simulink model "Model3Dpyhton"  (R2020a)
settings: Solver=VariableStepAuto  StartTime=0.0  StopTime=inf  FixedStep=0.2  RelTol=1e-3
model workspace (MAT data in the model file):
  VEH.Mass = 1181
  VEH.StaticNormalFrontLoad.FR = 264.666666667
  VEH.StaticNormalFrontLoad.FL = 264.666666667
  VEH.StaticNormalRearLoad.RR = 322
  VEH.StaticNormalRearLoad.RL = 322
  VEH.WheelBase = 3.075
  VEH.FrontAxlePositionfromCG = 1.515
  VEH.RearAxlePositionfromCG = 1.504
  VEH.HeightCG = 0.134
  VEH.FrontalArea = 2.11
  VEH.DragCoefficient = 0.33
  VEH.NumberOfWheelsPerAxle = 2
  VEH.Thread.FR = 1.705
  VEH.Thread.RR = 1.705
  VEH.PitchMomentInertia = 1922.66666667
  VEH.RollMomentInertia = 432.333333333
  VEH.YawMomentInertia = 2066
  VEH.SteeringRatio = 18
  VEH.TrackWidth = 1.922
  VEH.SprungMass = 1096.72266667
  VEH.InitialLongPosition = 0
  VEH.InitialLatPosition = 3.125
  VEH.InitialVertPosition = 0.0111
  VEH.InitialRollAngle = 0
  VEH.InitialPitchAngle = -0.000732
  VEH.InitialYawAngle = 0
  VEH.InitialLongVel = 0
  VEH.InitialLatVel = 0
  VEH.InitialVertVel = 0
  VEH.InitialRollRate = 0
  VEH.InitialPitchRate = 0
  VEH.InitialYawRate = 0
  color.orange = [1 0.6 0]
  color.red = [1 0.2 0]
  color.dgreen = [0 0.4 0]
  color.green = [0 0.6 0]
  color.lgreen = [0 0.8 0]
  color.dblue = [0 0.2 1]
  color.blue = [0.2 0.6 1]
  color.lblue = [0.4 0.8 1]
  color.brown = [0.4 0.2 0]
  color.lbrown = [0.8 0.4 0]
  color.yellow = [1 0.8 0]
  color.lyellow = [1 1 0]
  color.black = [0 0 0]
  color.white = [1 1 1]
  color.dgrey = [0.3 0.3 0.3]
  color.grey = [0.5 0.5 0.5]
  color.lgrey = [0.7 0.7 0.7]
  color.vlgrey = [0.9 0.9 0.9]
  cosAngle = 1
  density.wood = 650
  density.plastic = 920
  density.water = 1000
  density.aluminum = 2700
  density.steel = 7800
  density.titanium = 4500
  density.brass = 8600
  dwb.knuckle.height = 43
  dwb.knuckle.length = 8
  dwb.knuckle.thickness = 1
  dwb.knuckle.wheelattachprojwidth = 2.5
  dwb.knuckle.wheelattachprojheight = 8
  dwb.knuckle.wishboneconnectorwidth = 10
  dwb.knuckle.driveshaftradius = 2.5
  dwb.knuckle.driveshaftheight = 6
  dwb.knuckle.chamferradius = 0.25
  dwb.knuckle.transitionradius = 2
  dwb.knuckle.density = 2700
  dwb.knuckle.color = [0.3 0.3 0.3]
  dwb.knuckle.ball.radius = 1
  dwb.knuckle.pin.radius = 0.5
  dwb.knuckle.pin.height = 3
  dwb.knuckle.steerarm.length = 20
  dwb.knuckle.steerarm.width = 2
  dwb.knuckle.steerarm.thickness = 1
  dwb.knuckle.steerarm.forkheight = 13
  dwb.knuckle.steerarm.forklength = 4
  dwb.knuckle.steerarm.forkoffset = 3
  dwb.knuckle.pinradius = 0.25
  dwb.uwb.longlength = 25
  dwb.uwb.shortlength = 15
  dwb.uwb.wheellinklength = 5
  dwb.uwb.wheellinkwidth = 5
  dwb.uwb.width = 25
  dwb.uwb.thickness = 2
  dwb.uwb.baseradius = 8
  dwb.uwb.basearcoffset = 5
  dwb.uwb.density = 2700
  dwb.uwb.color = [0.3 0.2 0]
  dwb.uwb.bracket.length = 4
  dwb.uwb.bracket.radius = 0.75
  dwb.uwb.socket.radius = 2
  dwb.uwb.socket.height = 1.4
  dwb.uwb.socket.ballradius = 1
  dwb.uwb.socket.offset = 3
  dwb.lwb.longlength = 36
  dwb.lwb.shortlength = 25
  dwb.lwb.wheellinklength = 5
  dwb.lwb.wheellinkwidth = 5
  dwb.lwb.width = 14.75
  dwb.lwb.thickness = 2
  dwb.lwb.baseradius = 2.875
  dwb.lwb.basearcoffset = 15
  dwb.lwb.density = 2700
  dwb.lwb.color = [0.654901960784 0.423529411765 0.203921568627]
  dwb.lwb.bracket.length = 4
  dwb.lwb.bracket.radius = 0.75
  dwb.lwb.socket.radius = 2
  dwb.lwb.socket.height = 1.4
  dwb.lwb.socket.holeradius = 1
  dwb.lwb.socket.holeoffset = 3.0625
  dwb.lwb.damperbracket.offset = 10
  dwb.lwb.damperbracket.width = 4
  dwb.lwb.damperbracket.length = 4
  dwb.lwb.damperbracket.thickness = 1
  dwb.lwb.damperbracket.spacing = 1.5
  dwb.lwb.damperbracket.holeradius = 1
  dwb.springdamp.k = 100000
  dwb.springdamp.b = 11000
  dwb.springdamp.length0 = 18.5
  dwb.springdamp.density = 2700
  dwb.springdamp.cylinder.length = 22
  dwb.springdamp.cylinder.innerradius = 2
  dwb.springdamp.cylinder.outerradius = 3
  dwb.springdamp.cylinder.color = [0.9 0.7 0.2]
  dwb.springdamp.piston.length = 16
  dwb.springdamp.piston.color = [0.3 0.2 0]
  dwb.springdamp.chamferradius = 0.3
  dwb.springdamp.bracket.length = 6
  dwb.springdamp.bracket.width = 4
  dwb.springdamp.bracket.thickness = 1
  dwb.springdamp.bracket.holeradius = 0.75
  dwb.chassis.frame.longlength = 100
  dwb.chassis.frame.shortlength = 75
  dwb.chassis.frame.height = 40
  dwb.chassis.frame.cornerradius = 2
  dwb.chassis.frame.thickness = 2
  dwb.chassis.frame.barthickness = 5
  dwb.chassis.frame.density = 2700
  dwb.chassis.frame.color = [1 0.549019607843 0]
  dwb.chassis.upperlink.length = 30
  dwb.chassis.upperlink.outerradius = 1.5
  dwb.chassis.upperlink.innerradius = 0.75
  dwb.chassis.upperlink.wishboneslotlength = 5.5
  dwb.chassis.upperlink.springdamperslotlength = 3
  dwb.chassis.upperlink.wishboneseparation = 20.5
  dwb.chassis.upperlink.wishboneoffset = 0
  dwb.chassis.upperlink.chamferradius = 0.2
  dwb.chassis.upperlink.density = 2700
  dwb.chassis.upperlink.color = [1 0.549019607843 0]
  dwb.chassis.lowerlink.length = 30
  dwb.chassis.lowerlink.outerradius = 1.5
  dwb.chassis.lowerlink.innerradius = 0.75
  dwb.chassis.lowerlink.wishboneslotlength = 5.5
  dwb.chassis.lowerlink.wishboneseparation = 10.25
  dwb.chassis.lowerlink.wishboneoffset = 5.125
  dwb.chassis.lowerlink.chamferradius = 0.2
  dwb.chassis.lowerlink.density = 2700
  dwb.chassis.lowerlink.color = [1 0.549019607843 0]
  dwb.chassis.steering.bracket.length = 4
  dwb.chassis.steering.bracket.width = 4
  dwb.chassis.steering.bracket.thickness = 4
  dwb.chassis.steering.bracket.holelength = 2
  dwb.chassis.steering.bracket.holewidth = 2
  dwb.chassis.steering.bracket.chamferradius = 0.5
  dwb.chassis.steering.bracket.density = 2700
  dwb.chassis.steering.bracket.color = [1 0.549019607843 0]
  dwb.chassis.steering.tierod.rod.length = 16.5
  dwb.chassis.steering.tierod.rod.radius = 1.25
  dwb.chassis.steering.tierod.rod.chamferradius = 0.25
  dwb.chassis.steering.tierod.rod.color = [0.9 0.7 0.2]
  dwb.chassis.steering.tierod.bracket.length = 3
  dwb.chassis.steering.tierod.bracket.width = 2
  dwb.chassis.steering.tierod.bracket.thickness = 0.5
  dwb.chassis.steering.tierod.bracket.flangespacing = 0.75
  dwb.chassis.steering.tierod.bracket.socketradius = 0.75
  dwb.chassis.steering.tierod.bracket.ballradius = 0.5
  dwb.chassis.steering.tierod.bracket.holeradius = 0.3
  dwb.chassis.steering.tierod.density = 2700
  dwb.chassis.steering.tierod.ballcolor = [0.3 0.2 0]
  dwb.chassis.steering.rack.rod.length = 120
  dwb.chassis.steering.rack.rod.width = 2
  dwb.chassis.steering.rack.rod.height = 2
  dwb.chassis.steering.rack.rod.bracketdistance = 70
  dwb.chassis.steering.rack.rod.chamferradius = 0.5
  dwb.chassis.steering.rack.bracket.length = 4
  dwb.chassis.steering.rack.bracket.width = 2
  dwb.chassis.steering.rack.bracket.thickness = 0.5
  dwb.chassis.steering.rack.bracket.holeradius = 0.5
  dwb.chassis.steering.rack.density = 2700
  dwb.chassis.steering.rack.color = [0.3 0.2 0]
  mp.knuckle.springdamperangle = 30
  mp.knuckle.balldiameter = 1
  mp.knuckle.hublength = 15
  mp.knuckle.density = 2700
  mp.knuckle.color = [0.5 0.5 0.5]
  mp.springdamp.k = 50000
  mp.springdamp.b = 1500
  mp.springdamp.length0 = 15
  mp.springdamp.density = 2700
  mp.springdamp.cylinder.length = 22
  mp.springdamp.cylinder.innerradius = 2
  mp.springdamp.cylinder.outerradius = 3
  mp.springdamp.cylinder.color = [0.9 0.7 0.2]
  mp.springdamp.piston.length = 15
  mp.springdamp.piston.color = [0.55 0.35 0.17]
  mp.springdamp.chamferradius = 0.3
  mp.springdamp.bracket.length = 4
  mp.springdamp.bracket.width = 4
  mp.springdamp.bracket.thickness = 1
  mp.springdamp.bracket.holeradius = 0.75
  mp.wb.longlength = 20
  mp.wb.shortlength = 10
  mp.wb.wheellinklength = 5
  mp.wb.wheellinkwidth = 5
  mp.wb.width = 14.75
  mp.wb.thickness = 2
  mp.wb.baseradius = 2.875
  mp.wb.basearcoffset = 5
  mp.wb.density = 2700
  mp.wb.color = [0.5 0.5 0.5]
  mp.wb.bracket.length = 4
  mp.wb.bracket.radius = 1
  mp.wb.socket.radius = 2
  mp.wb.socket.height = 1.4
  mp.wb.socket.ballradius = 1
  mp.wb.socket.offset = 3
  mp.chassis.frame.longlength = 125
  mp.chassis.frame.shortlength = 100
  mp.chassis.frame.height = 50
  mp.chassis.frame.cornerradius = 2
  mp.chassis.frame.thickness = 2
  mp.chassis.frame.barthickness = 5
  mp.chassis.frame.density = 2700
  mp.chassis.frame.color = [1 0.549019607843 0]
  mp.chassis.upperlink.length = 30
  mp.chassis.upperlink.outerradius = 1.5
  mp.chassis.upperlink.innerradius = 0.75
  mp.chassis.upperlink.springdamperslotlength = 3
  mp.chassis.upperlink.springdamperoffset = 8
  mp.chassis.upperlink.chamferradius = 0.2
  mp.chassis.upperlink.density = 2700
  mp.chassis.upperlink.color = [1 0.549019607843 0]
  mp.chassis.lowerlink.length = 30
  mp.chassis.lowerlink.outerradius = 1.5
  mp.chassis.lowerlink.innerradius = 0.75
  mp.chassis.lowerlink.wishboneslotlength = 5.5
  mp.chassis.lowerlink.wishboneseparation = 10.25
  mp.chassis.lowerlink.wishboneoffset = 3.125
  mp.chassis.lowerlink.chamferradius = 0.2
  mp.chassis.lowerlink.density = 2700
  mp.chassis.lowerlink.color = [1 0.549019607843 0]
  number1 = 5
  platform.cylinder.outerradius = 12
  platform.cylinder.innerradius = 10
  platform.cylinder.flangeradius = 20
  platform.cylinder.flangethickness = 2
  platform.cylinder.height = 40
  platform.cylinder.color = [0.3 0.3 0.3]
  platform.cylinder.leftlocation = [-80 -25 0]
  platform.cylinder.rightlocation = [80 -25 0]
  platform.piston.innerradius = 8
  platform.piston.height = 60
  platform.piston.color = [0.6 0.6 0.6]
  platform.base.length = 40
  platform.base.width = 40
  platform.base.thickness = 3
  platform.base.color = [0.6 0.6 0.6]
  platform.controller.k = 10000
  platform.controller.kd = 100
  platform.density = 2700
  pr.knuckle.height = 43
  pr.knuckle.length = 8
  pr.knuckle.thickness = 1
  pr.knuckle.wheelattachprojwidth = 2.5
  pr.knuckle.wheelattachprojheight = 8
  pr.knuckle.wishboneconnectorwidth = 10
  pr.knuckle.driveshaftradius = 2.5
  pr.knuckle.driveshaftheight = 6
  pr.knuckle.chamferradius = 0.25
  pr.knuckle.transitionradius = 2
  pr.knuckle.density = 2700
  pr.knuckle.color = [0.3 0.3 0.3]
  pr.knuckle.ball.radius = 1
  pr.knuckle.pin.radius = 0.5
  pr.knuckle.pin.height = 3
  pr.knuckle.steerarm.length = 20
  pr.knuckle.steerarm.width = 2
  pr.knuckle.steerarm.thickness = 1
  pr.knuckle.steerarm.forkheight = 13
  pr.knuckle.steerarm.forklength = 4
  pr.knuckle.steerarm.forkoffset = 3
  pr.knuckle.pinradius = 0.25
  pr.uwb.longlength = 25
  pr.uwb.shortlength = 15
  pr.uwb.wheellinklength = 5
  pr.uwb.wheellinkwidth = 5
  pr.uwb.width = 25
  pr.uwb.thickness = 2
  pr.uwb.baseradius = 8
  pr.uwb.basearcoffset = 5
  pr.uwb.density = 2700
  pr.uwb.color = [0.3 0.2 0]
  pr.uwb.bracket.length = 4
  pr.uwb.bracket.radius = 0.75
  pr.uwb.socket.radius = 2
  pr.uwb.socket.height = 1.4
  pr.uwb.socket.ballradius = 1
  pr.uwb.socket.offset = 3
  pr.lwb.longlength = 36
  pr.lwb.shortlength = 25
  pr.lwb.wheellinklength = 5
  pr.lwb.wheellinkwidth = 5
  pr.lwb.width = 14.75
  pr.lwb.thickness = 2
  pr.lwb.baseradius = 2.875
  pr.lwb.basearcoffset = 15
  pr.lwb.density = 2700
  pr.lwb.color = [0.654901960784 0.423529411765 0.203921568627]
  pr.lwb.bracket.length = 4
  pr.lwb.bracket.radius = 0.75
  pr.lwb.socket.radius = 2
  pr.lwb.socket.height = 1.4
  pr.lwb.socket.holeradius = 1
  pr.lwb.socket.holeoffset = 3.0625
  pr.lwb.damperbracket.offset = 10
  pr.lwb.damperbracket.width = 4
  pr.lwb.damperbracket.length = 4
  pr.lwb.damperbracket.thickness = 1
  pr.lwb.damperbracket.spacing = 1.5
  pr.lwb.damperbracket.holeradius = 1
  pr.pr.radius = 1
  pr.pr.length = 30
  pr.pr.bracket.length = 4
  pr.pr.bracket.width = 4
  pr.pr.bracket.thickness = 1
  pr.pr.bracket.holeradius = 0.75
  pr.pr.density = 2700
  pr.pr.cylinder.color = [0.9 0.7 0.2]
  pr.pr.piston.color = [0.55 0.35 0.17]
  pr.rocker.armlength = 10
  pr.rocker.motionratio = 1
  pr.rocker.thickness = 3
  pr.rocker.density = 7800
  pr.rocker.color = [0.5 0.5 0.5]
  pr.springdamp.k = 200000
  pr.springdamp.b = 3000
  pr.springdamp.length0 = 15
  pr.springdamp.density = 2700
  pr.springdamp.cylinder.length = 15
  pr.springdamp.cylinder.innerradius = 2
  pr.springdamp.cylinder.outerradius = 3
  pr.springdamp.cylinder.color = [0.9 0.7 0.2]
  pr.springdamp.piston.length = 10
  pr.springdamp.piston.color = [0.55 0.35 0.17]
  pr.springdamp.chamferradius = 0.3
  pr.springdamp.bracket.length = 4
  pr.springdamp.bracket.width = 4
  pr.springdamp.bracket.thickness = 1
  pr.springdamp.bracket.holeradius = 0.75
  pr.chassis.frame.pushrodoffset = 25
  pr.chassis.frame.longlength = 100
  pr.chassis.frame.shortlength = 75
  pr.chassis.frame.height = 40
  pr.chassis.frame.cornerradius = 2
  pr.chassis.frame.thickness = 2
  pr.chassis.frame.barthickness = 5
  pr.chassis.frame.density = 2700
  pr.chassis.frame.color = [1 0.549019607843 0]
  pr.chassis.upperlink.length = 30
  pr.chassis.upperlink.outerradius = 1.5
  pr.chassis.upperlink.innerradius = 0.75
  pr.chassis.upperlink.wishboneslotlength = 5.5
  pr.chassis.upperlink.springdamperslotlength = 3
  pr.chassis.upperlink.wishboneseparation = 20.5
  pr.chassis.upperlink.wishboneoffset = 0
  pr.chassis.upperlink.chamferradius = 0.2
  pr.chassis.upperlink.density = 2700
  pr.chassis.upperlink.color = [1 0.549019607843 0]
  pr.chassis.lowerlink.length = 30
  pr.chassis.lowerlink.outerradius = 1.5
  pr.chassis.lowerlink.innerradius = 0.75
  pr.chassis.lowerlink.wishboneslotlength = 5.5
  pr.chassis.lowerlink.wishboneseparation = 10.25
  pr.chassis.lowerlink.wishboneoffset = 5.125
  pr.chassis.lowerlink.chamferradius = 0.2
  pr.chassis.lowerlink.density = 2700
  pr.chassis.lowerlink.color = [1 0.549019607843 0]
  pr.chassis.lowerlink2.length = 30
  pr.chassis.lowerlink2.outerradius = 1.5
  pr.chassis.lowerlink2.innerradius = 0.75
  pr.chassis.lowerlink2.springdamperslotlength = 3
  pr.chassis.lowerlink2.springdamperoffset = 0
  pr.chassis.lowerlink2.chamferradius = 0.2
  pr.chassis.lowerlink2.density = 2700
  pr.chassis.lowerlink2.color = [1 0.549019607843 0]
  pr.chassis.steering.bracket.length = 4
  pr.chassis.steering.bracket.width = 4
  pr.chassis.steering.bracket.thickness = 4
  pr.chassis.steering.bracket.holelength = 2
  pr.chassis.steering.bracket.holewidth = 2
  pr.chassis.steering.bracket.chamferradius = 0.5
  pr.chassis.steering.bracket.density = 2700
  pr.chassis.steering.bracket.color = [1 0.549019607843 0]
  pr.chassis.steering.tierod.rod.length = 16.5
  pr.chassis.steering.tierod.rod.radius = 1.25
  pr.chassis.steering.tierod.rod.chamferradius = 0.25
  pr.chassis.steering.tierod.rod.color = [0.9 0.7 0.2]
  pr.chassis.steering.tierod.bracket.length = 3
  pr.chassis.steering.tierod.bracket.width = 2
  pr.chassis.steering.tierod.bracket.thickness = 0.5
  pr.chassis.steering.tierod.bracket.flangespacing = 0.75
  pr.chassis.steering.tierod.bracket.socketradius = 0.75
  pr.chassis.steering.tierod.bracket.ballradius = 0.5
  pr.chassis.steering.tierod.bracket.holeradius = 0.3
  pr.chassis.steering.tierod.density = 2700
  pr.chassis.steering.tierod.ballcolor = [0.3 0.2 0]
  pr.chassis.steering.rack.rod.length = 120
  pr.chassis.steering.rack.rod.width = 2
  pr.chassis.steering.rack.rod.height = 2
  pr.chassis.steering.rack.rod.bracketdistance = 70
  pr.chassis.steering.rack.rod.chamferradius = 0.5
  pr.chassis.steering.rack.bracket.length = 4
  pr.chassis.steering.rack.bracket.width = 2
  pr.chassis.steering.rack.bracket.thickness = 0.5
  pr.chassis.steering.rack.bracket.holeradius = 0.5
  pr.chassis.steering.rack.density = 2700
  pr.chassis.steering.rack.color = [0.3 0.2 0]
  sinAngle = 1
  wheel.tire.innerradius = 25
  wheel.tire.outerradius = 30
  wheel.tire.width = 15
  wheel.tire.chamferradius = 1
  wheel.tire.density = 1000
  wheel.tire.color = [0 0 0]
  wheel.hub.radius = 5
  wheel.hub.outerradius = 23
  wheel.hub.numspokes = 5
  wheel.hub.spokethickness = 1
  wheel.hub.width = 11
  wheel.hub.density = 2700
  wheel.hub.color = [0.5 0.5 0.5]
  wheel.shaft.length = 6
  wheel.shaft.radius = 2
  wheel.disc.radius = 10
  wheel.disc.thickness = 1
libraries: autolibutils x4, sim3dlib x3, autolibshared x2, simulink x1, vdynlib x1, vehdynlibsteering x1, instrumentlib x1
(part 1 of 3)
settings Model: SimulationMode=accelerator  PacingRate=1000  Creator=Ishmael  LastModifiedBy=eduar
settings SolverCC: ZeroCrossAlgorithm=Adaptive  AlgebraicLoopSolver=LineSearch  DecoupledContinuousIntegration=on  MinimalZcImpactIntegration=on
settings DataIOCC: SaveFormat=Array  SaveOutput=off  ReturnWorkspaceOutputsName=FrameCopy_spidata
settings OptimizationCC: OptimizeBlockIOStorage=off  EnhancedBackFolding=on  PassReuseOutputArgsThreshold=0  MaxStackSize=64  OptimizeDataStoreBuffers=off  BusAssignmentInplaceUpdate=off
settings DebuggingCC: ReadBeforeWriteMsg=DisableAll  WriteAfterWriteMsg=DisableAll  WriteAfterReadMsg=DisableAll  IgnoredZcDiagnostic=none  MultiTaskDSMMsg=none  ParameterTunabilityLossMsg=error  SFUnexpectedBacktrackingDiag=warning  SFNoUnconditionalDefaultTransitionDiag=warning
settings HardwareCC: ProdBitPerPointer=32  ProdBitPerSizeT=32  ProdBitPerPtrDiffT=32  ProdLargestAtomicFloat=None  ProdIntDivRoundTo=Undefined  ProdEndianess=Unspecified  ProdWordSize=32  ProdHWDeviceType=Custom Processor->Custom Processor
settings ModelReferenceCC: PropagateSignalLabelsOutOfModel=off
settings SFSimCC: SFSimEcho=off  SimAnalyzeCustomCode=on  MATLABDynamicMemAlloc=off  CustomCodeUndefinedFunction=UseInterfaceOnly
settings RTWCC: Description=Generic Real-Time Target  GenerateReport=on  BuildConfiguration=Debug  LaunchReport=on
settings CodeAppCC: ForceParamTrailComments=on  OperatorAnnotations=on  MATLABSourceComments=on  EnableCustomComments=on
settings GRTTargetCC: TargetLangStandard=C89/C90 (ANSI)  CombineSignalStateStructs=on  MultiInstanceERTCode=on  CodeInterfacePackaging=Reusable function  SupportVariableSizeSignals=on  GenerateAllocFcn=on  MultiInstanceErrorCode=Warning
settings ConfigComp: CovScope=ReferencedModels  CovIncludeTopModel=off
settings SimscapeCC: SimscapeNormalizeSystem=off
settings DiagnosticsConfigSet: SimMechanicsUnconnectedFramePorts=none  SimMechanicsRigidlyBoundBlock=none  SimMechanicsUnsatisfiedHighPriorityTargets=none
settings ExplorerConfigSet: InternalSimMechanicsExplorerSettings="<ExplorerConfiguration><canonicalview>default</canonicalview><AnimationSetting><BasePlaybackSpeed>1.0</BasePlaybackSpeed><PlaybackSpeedFactor>1.0</PlaybackSpeedFactor></AnimationSetting><TilePanel><TileInfo><Tiles Columns=\"1\" Count=\"1\" Rows=\"1\"><Column Weight=\"1\"/><Row Weight=\"1\"/><Tile Height=\"1\" Width=\"1\" X=\"0\" Y=\"0\"/></Tiles></TileInfo><SceneInfo><SceneViewer><BGColor><R>0.60000002384185791</R><G>0.60000002384185791</G><B>0.60000002384185791</B></BGColor><Camera><DoPerspective>on</DoPerspective><Position><X>3.28112680635967308e-15</X><Y>-7.5</Y><Z>3.35000000000000098</Z></Position><Center><X>1.77635683940025046e-15</X><Y>-2.22044604925031308e-16</Y><Z>0.349999999999999978</Z></Center><Up><X>-5.35215233261039919e-17</X><Y>9.30804934765350176e-17</Y><Z>1</Z></Up><ViewLimDist>1</ViewLimDist><YLim>0.466307658154998583</YLim><XLim>0.595525442944937922</XLim></Camera></SceneViewer></SceneInfo></TilePanel><MechEditorPanel><Cameras><Camera><Id>Camera1</Id><Value><Name>Camera1</Name><NativeCamera><PositionTrackingFeature>Model.Model.Subsystem.Cameras.Follower_Camera_Transform.F</PositionTrackingFeature><CenterTrackingFeature>Model.Model.Subsystem.Cameras.Follower_Camera_Transform.B</CenterTrackingFeature><UpVectorTrackingFeature>Model.Model.Subsystem.Cameras.Follower_Camera_Transform.B</UpVectorTrackingFeature><CenterTrackingOrigin>on</CenterTrackingOrigin><UpVectorTrackingDirection>+Z</UpVectorTrackingDirection></NativeCamera></Value></Camera></Cameras><GfxPanelCameraMap><MapElement CameraMLId=\"Camera1\" GfxPanelIndex=\"0\"/></GfxPanelCameraMap><VideoCreator><PlaybackSpeedRatio>1.0</PlaybackSpeedRatio><FrameRate>30</FrameRate><VideoFormat>Motion JPEG AVI</VideoFormat><FrameSize>auto</FrameSize></VideoCreator></MechEditorPanel></ExplorerConfiguration>"

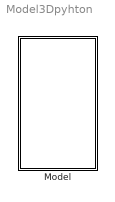
== system Model3Dpyhton ==
  Model : Subsystem

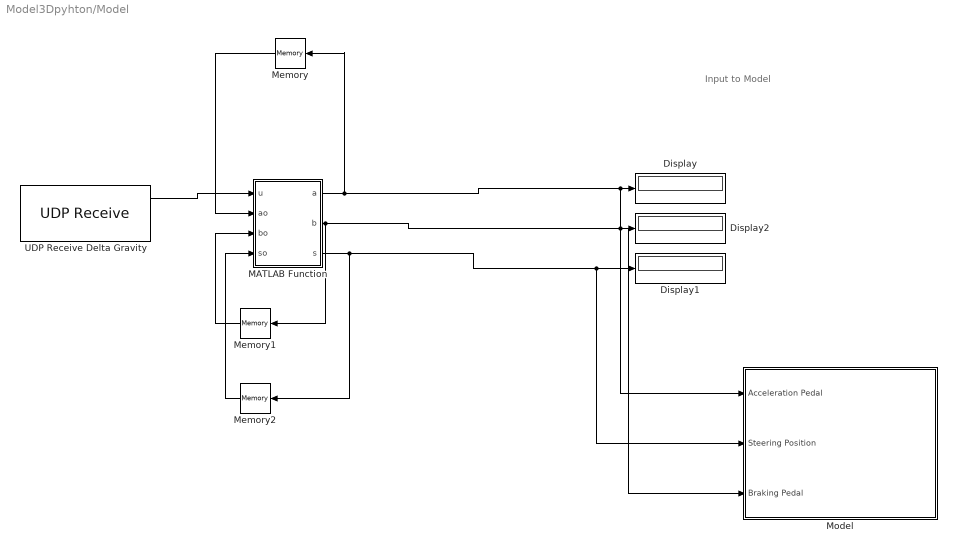
== system Model3Dpyhton/Model ==
  note: Input to Model
  Display : Display
  Display1 : Display
  Display2 : Display
  MATLAB Function : MATLAB Function  TreatAsAtomicUnit=on
  Memory : Memory
  Memory1 : Memory
  Memory2 : Memory
  Model : Subsystem
  UDP Receive Delta Gravity : instrumentlib/UDP Receive  Host=localhost  Port=9090  LocalPort=54320  EnablePortSharing=off  GetLatestData=on  DataSize="[1  1]"  DataType=ASCII  ASCIIFormatting=%d  Terminator=LF  ByteOrder=LittleEndian  EnableBlockingMode=off  Timeout=10  SampleTime=0.01  LocalAddress=localhost
  wires:
  MATLAB Function/2(b) -> Memory1/1, Model/3(Braking Pedal), Display2/1
  UDP Receive Delta Gravity/1 -> MATLAB Function/1(u)
  MATLAB Function/3(s) -> Memory2/1, Display1/1, Model/2(Steering Position)
  MATLAB Function/1(a) -> Memory/1, Model/1(Acceleration Pedal), Display/1
  Memory1/1 -> MATLAB Function/3(bo)
  Memory2/1 -> MATLAB Function/4(so)
  Memory/1 -> MATLAB Function/2(ao)

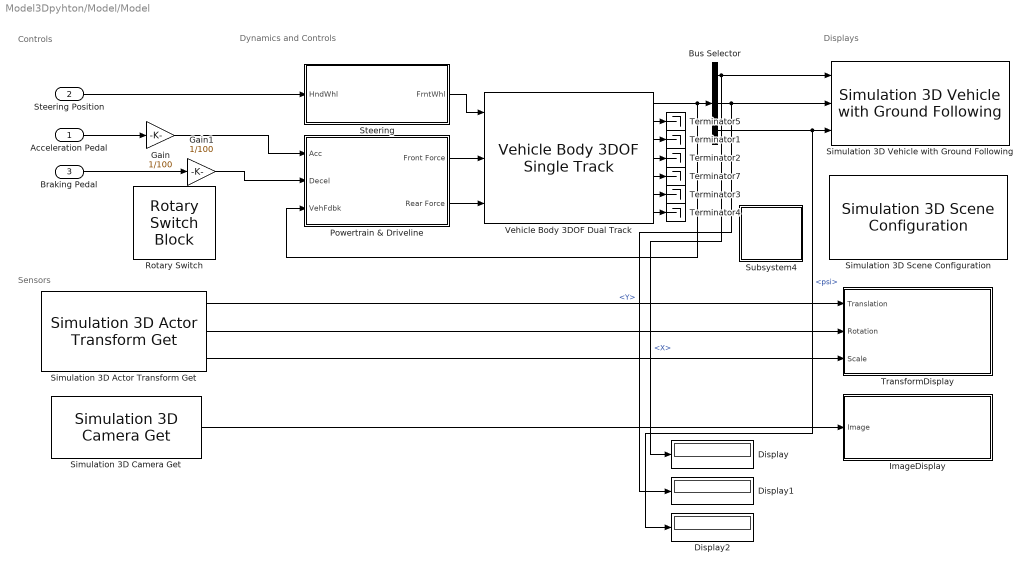
== system Model3Dpyhton/Model/Model ==
  note: Sensors
  note: Displays
  note: Controls
  note: Dynamics and Controls
  Acceleration Pedal : Inport
  Steering Position : Inport  Port=2
  Braking Pedal : Inport  Port=3
  Bus Selector : BusSelector  OutputSignals=InertFrm.Geom.Disp.X,InertFrm.Geom.Disp.Y,InertFrm.Cg.Ang.psi
  Display : Display
  Display1 : Display
  Display2 : Display
  Gain : Gain  Gain=1/100
  Gain1 : Gain  Gain=1/100
  ImageDisplay : Subsystem
  Powertrain & Driveline : Subsystem
      mask Display: image('vdbslibpt.png');
  Rotary Switch : RotarySwitchBlock  LabelPosition=Bottom
      settings: Values={{'R', 'N', 'D'}, [-1 0 1]}
  Simulation 3D Actor Transform Get : sim3dlib/Simulation 3D Actor Transform Get  Priority=1  ActorTag=GolfCart  NumberOfParts=5  CustNumOfParts=3  Ts=-1  aMode=2
      settings: SourceProductBaseCode=DR,VE
  Simulation 3D Camera Get : sim3dlib/Simulation 3D Camera Get  Priority=2  sensorTag=Sim3dSensor1  sensorId=1  sensorName=Sim3dSensor1  vehTagList={'GolfCart';'Scene Origin'}  vehTag=GolfCart  mountLoc=Roof center  offsetFlag=off  tmountOffset=[0, 0, 0]  rmountOffset=[0, 0, 0]  HorizontalResolution=1024  VerticalResolution=768  HorizontalFOV=90  SampleTime=.02  mountPoint=[-0.25 0 1.57000005245209]  mountOrientation=[0 0 0]  aMode=2  ID=1
      settings: SourceProductBaseCode=DR,VE
  Simulation 3D Scene Configuration : sim3dlib/Simulation 3D Scene Configuration  Priority=1  ProjectFormat=Default Scenes  SceneDesc=Straight road  ProjectName=VehicleSimulation.exe  ScenePath=/Game/Maps/HwStrght  vehTagList={'GolfCart';'Scene Origin'}  vehTag=GolfCart  OpVisEn=off  Ts=.02  EnableWindow=on  sensorTag=MainCamera1  sensorId=1  sensorName=MainCamera1  mountLoc=Origin  offsetFlag=off  tmountOffset=[0, 0, 0]  rmountOffset=[0, 0, 0]  HorizontalResolution=1280  VerticalResolution=720  HorizontalFOV=60  mountPoint=[0 0 0]  mountOrientation=[0 0 0]  aMode=2  ID=1
      settings: SourceProductBaseCode=DR,VE
  Simulation 3D Vehicle with Ground Following : vdynlib/Vehicle Scenarios/Sim3D/Sim3D Vehicle/Components/Simulation 3D Vehicle with Ground Following  Priority=-1  PassVehMesh=Muscle car  VehColor=Silver  InitialPos=[60,1, 0]  InitialRot=[0, 0, 0]  ActorName=GolfCart  SampleTime=-1  ActorType=SimulinkVehicle  ID=C  aMode=2  ActorTag=GolfCart  CoordinateScheme=SAE
      settings: SourceProductBaseCode=VE
  Steering : Subsystem
      mask Display: image('vdbslibsteer.png');
  Subsystem4 : Subsystem
      settings: OpenFcn=eval('vdynblkshelp(''vdynblksscenecameraray'')');
      mask Display: disp('Help')
  Terminator{1..5,7} (6 alike) : Terminator
  TransformDisplay : Subsystem
  Vehicle Body 3DOF Dual Track : autolibshared/Vehicle Body 3DOF Single Track  trackMode=Dual  inputMode=External longitudinal forces  frontSteerMode=on  rearSteerMode=off  windMode=off  muMode=off  extFMode=off  extMMode=off  extXo=off  extpsio=off  extxdoto=off  extro=off  extYo=off  extTamb=off  extydoto=off  aMode=2  NF=2  NR=2  m=400  a=1.4  b=1.6  h=0.35  X_o=0  xdot_o=0  CalphaMode=off  sigmaMode=on  d=0  w=[1.4,1.4]  Cy_f=12e3  Cy_r=11e3  sigma_f=.1  sigma_r=.1  alpha_f_brk=[-.1 .1]  Cy_f_data=[-9e3 9e3]  alpha_r_brk=[-.1 .1]  Cy_r_data=[-9e3 9e3]  Y_o=3.15  ydot_o=0  Izz=2000  psi_o=0  r_o=0  Af=2  Cd=.3  Cl=.1  Cpm=.1  beta_w=[0:0.01:0.3]  Cs=[0:0.03:0.9]  Cym=[0:0.01:0.3]  Pabs=101325  Tair=273  g=9.81  mu=1  xdot_tol=.1  Fznom=5000  Fxtire_sat=7e4  Fytire_sat=7e4  longOff=0  latOff=0  vertOff=0  wrapAng=off
      settings: SourceProductBaseCode=PW,MT,VE,VP
  wires:
  Steering/1(FrntWhl) -> Vehicle Body 3DOF Dual Track/1
  Simulation 3D Camera Get/1 -> ImageDisplay/1(Image)
  Vehicle Body 3DOF Dual Track/5 -> Terminator7/1
  Steering Position/1 -> Steering/1(HndWhl)
  Bus Selector/3 -> Display2/1, Simulation 3D Vehicle with Ground Following/3  "<psi>"
  Simulation 3D Actor Transform Get/3 -> TransformDisplay/3(Scale)
  Vehicle Body 3DOF Dual Track/2 -> Terminator5/1
  Acceleration Pedal/1 -> Gain/1
  Powertrain & Driveline/2(Rear Force) -> Vehicle Body 3DOF Dual Track/3
  Braking Pedal/1 -> Gain1/1
  Vehicle Body 3DOF Dual Track/6 -> Terminator3/1
  Powertrain & Driveline/1(Front Force) -> Vehicle Body 3DOF Dual Track/2
  Vehicle Body 3DOF Dual Track/7 -> Terminator4/1
  Vehicle Body 3DOF Dual Track/1 -> Powertrain & Driveline/3(VehFdbk), Bus Selector/1
  Bus Selector/1 -> Display/1, Simulation 3D Vehicle with Ground Following/1  "<X>"
  Vehicle Body 3DOF Dual Track/4 -> Terminator2/1
  Bus Selector/2 -> Display1/1, Simulation 3D Vehicle with Ground Following/2  "<Y>"
  Simulation 3D Actor Transform Get/1 -> TransformDisplay/1(Translation)
  Simulation 3D Actor Transform Get/2 -> TransformDisplay/2(Rotation)
  Vehicle Body 3DOF Dual Track/3 -> Terminator1/1
  Gain/1 -> Powertrain & Driveline/1(Acc)
  Gain1/1 -> Powertrain & Driveline/2(Decel)

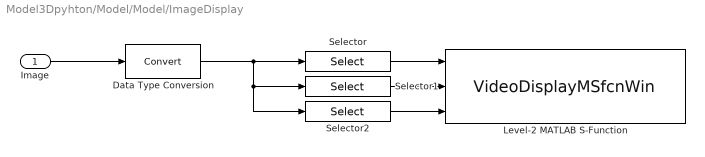
== system Model3Dpyhton/Model/Model/ImageDisplay ==
  Image : Inport
  Data Type Conversion : DataTypeConversion
  Level-2 MATLAB S-Function : M-S-Function  FunctionName=VideoDisplayMSfcnWin  Parameters=1
  Selector : Selector  NumberOfDimensions=3  InputPortWidth=3  IndexOptions=Select all,Select all,Index vector (dialog)  Indices=[1 3],1,1  OutputSizes=1,1,1
  Selector1 : Selector  NumberOfDimensions=3  InputPortWidth=3  IndexOptions=Select all,Select all,Index vector (dialog)  Indices=[1 3],1,2  OutputSizes=1,1,1
  Selector2 : Selector  NumberOfDimensions=3  InputPortWidth=3  IndexOptions=Select all,Select all,Index vector (dialog)  Indices=[1 3],1,3  OutputSizes=1,1,1
  wires:
  Data Type Conversion/1 -> Selector2/1, Selector1/1, Selector/1
  Image/1 -> Data Type Conversion/1
  Selector1/1 -> Level-2 MATLAB S-Function/2
  Selector2/1 -> Level-2 MATLAB S-Function/3
  Selector/1 -> Level-2 MATLAB S-Function/1

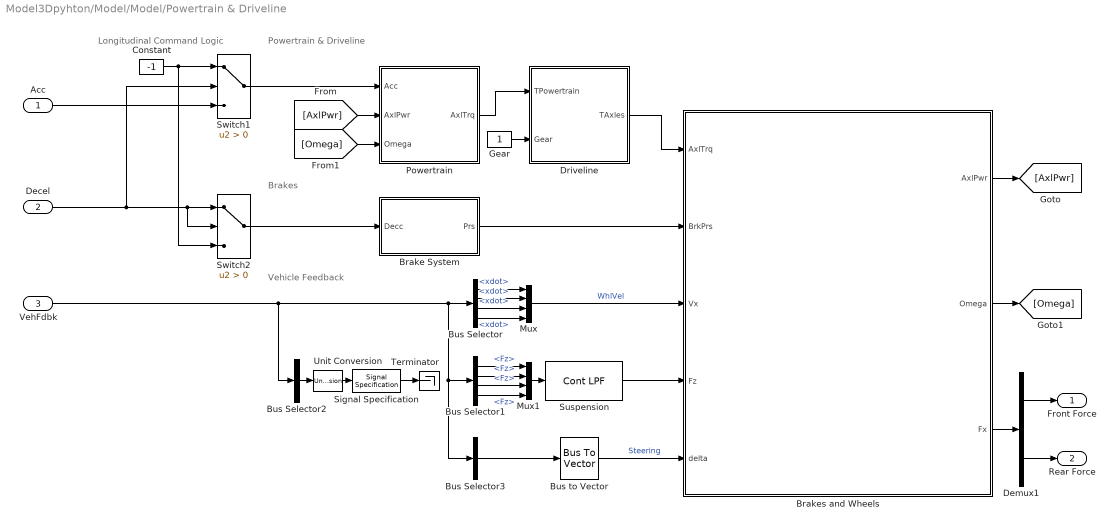
== system Model3Dpyhton/Model/Model/Powertrain & Driveline ==
  note: Longitudinal Command Logic
  note: Brakes
  note: Powertrain & Driveline
  note: Vehicle Feedback
  Acc : Inport
  Decel : Inport  Port=2
  VehFdbk : Inport  Port=3
  Brake System : Subsystem
  Brakes and Wheels : Subsystem  TreatAsAtomicUnit=on
      mask Display: image('vdbslibwhls.png');
  Bus Selector : BusSelector  OutputSignals=BdyFrm.FrntAxl.Lft.Vel.xdot,BdyFrm.FrntAxl.Rght.Vel.xdot,BdyFrm.RearAxl.Lft.Vel.xdot,BdyFrm.RearAxl.Rght.Vel.xdot
  Bus Selector1 : BusSelector  OutputSignals=BdyFrm.Forces.FrntAxl.Lft.Fz,BdyFrm.Forces.FrntAxl.Rght.Fz,BdyFrm.Forces.RearAxl.Lft.Fz,BdyFrm.Forces.RearAxl.Rght.Fz
  Bus Selector2 : BusSelector  OutputSignals=BdyFrm.Cg.Vel.xdot  OutputAsBus=on
  Bus Selector3 : BusSelector  OutputSignals=BdyFrm.FrntAxl.Steer.WhlAngFL,BdyFrm.FrntAxl.Steer.WhlAngFR,BdyFrm.RearAxl.Steer.WhlAngRL,BdyFrm.RearAxl.Steer.WhlAngRR  OutputAsBus=on
  Bus to Vector : BusToVector
  Constant : Constant  Value=-1
  Demux1 : Demux  Outputs=[2 2]
  Driveline : Subsystem  Variant=on  VariantControlMode=Label  VariantControl=Variant1  LabelModeActiveChoice=0
  Gear : Constant
  Mux : Mux
  Mux1 : Mux
  Powertrain : Subsystem
  Signal Specification : SignalSpecification  Unit=km/hr
  Suspension : autolibutils/Cont LPF  wc=10*pi*2  aMode=2
      settings: SourceProductBaseCode=PW,MT,VE,VP
  Switch1 : Switch  Criteria=u2 > Threshold
  Switch2 : Switch  Criteria=u2 > Threshold
  Terminator : Terminator
  Unit Conversion : UnitConversion
  Front Force : Outport  VectorParamsAs1DForOutWhenUnconnected=off
  Rear Force : Outport  Port=2  VectorParamsAs1DForOutWhenUnconnected=off
  wires:
  Decel/1 -> Switch1/2, Switch2/2, Switch2/1
  Acc/1 -> Switch1/3
  Constant/1 -> Switch2/3, Switch1/1
  Mux/1 -> Brakes and Wheels/3(Vx)  "WhlVel"
  VehFdbk/1 -> Bus Selector2/1, Bus Selector3/1, Bus Selector1/1, Bus Selector/1
  Demux1/1 -> Front Force/1
  Demux1/2 -> Rear Force/1
  Driveline/1(TAxles) -> Brakes and Wheels/1(AxlTrq)
  Brakes and Wheels/1(AxlPwr) -> [AxlPwr]
  Brakes and Wheels/3(Fx) -> Demux1/1
  Bus Selector3/1 -> Bus to Vector/1
  Bus to Vector/1 -> Brakes and Wheels/5(delta)  "Steering"
  Mux1/1 -> Suspension/1
  Suspension/1 -> Brakes and Wheels/4(Fz)
  Bus Selector/1 -> Mux/1  "<xdot>"
  Bus Selector/2 -> Mux/2  "<xdot>"
  Bus Selector/3 -> Mux/3  "<xdot>"
  Bus Selector/4 -> Mux/4  "<xdot>"
  Bus Selector1/1 -> Mux1/1  "<Fz>"
  Bus Selector1/2 -> Mux1/2  "<Fz>"
  Bus Selector1/3 -> Mux1/3  "<Fz>"
  Bus Selector1/4 -> Mux1/4  "<Fz>"
  Switch1/1 -> Powertrain/1(Acc)
  Powertrain/1(AxlTrq) -> Driveline/1(TPowertrain)
  Brakes and Wheels/2(Omega) -> [Omega]
  [AxlPwr] -> Powertrain/2(AxlPwr)
  [Omega] -> Powertrain/3(Omega)
  Switch2/1 -> Brake System/1(Decc)
  Brake System/1(Prs) -> Brakes and Wheels/2(BrkPrs)
  Bus Selector2/1 -> Unit Conversion/1
  Unit Conversion/1 -> Signal Specification/1
  Signal Specification/1 -> Terminator/1
  Gear/1 -> Driveline/2(Gear)

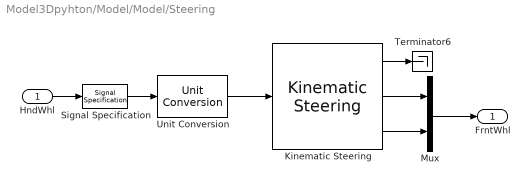
== system Model3Dpyhton/Model/Model/Steering ==
  HndWhl : Inport
  Kinematic Steering : vehdynlibsteering/Kinematic Steering  StrgType=Rack and pinion  StrgRatioType=Constant  Loc=Front  NrmlFctr=0.01  TrckWdth=1.4  WhlBase=1.524  Db=0  StrgRng=1.25*pi  StrgAngBpts="[-6.2832   -5.0265   -3.7699   -2.5133   -1.2566         0    1.2566    2.5133    3.7699    5.0265    6.2832]"  StrgRatioTbl=|  StrgRatio=100  StrgArmLngth=0.1  RckCsLngth=0.5  TieRodLngth=.4  D=0.2  PnnRadius=0.0057  PnnRadiusTbl="[0.0055    0.0055    0.0056    0.0057    0.0058    0.0057    0.0057    0.0057    0.0056    0.0055    0.0055]"  RodLngth=0.1  ParaArmLngth=0.9  aMode=2
      | [13.5000   13.3750   13.2500   13.1250   13.0000   13.0000   13.0000   13.1250   13.2500   13.3750   13.5000
      | ]
  Mux : Mux  Inputs=2
  Signal Specification : SignalSpecification  Unit=deg
  Terminator6 : Terminator
  Unit Conversion : UnitConversion
  FrntWhl : Outport  VectorParamsAs1DForOutWhenUnconnected=off
  wires:
  Signal Specification/1 -> Unit Conversion/1
  Kinematic Steering/1 -> Terminator6/1
  HndWhl/1 -> Signal Specification/1
  Kinematic Steering/2 -> Mux/1
  Kinematic Steering/3 -> Mux/2
  Unit Conversion/1 -> Kinematic Steering/1
  Mux/1 -> FrntWhl/1

== system Model3Dpyhton/Model/Model/Subsystem4 ==

== system Model3Dpyhton/Model/Model/TransformDisplay ==
  Translation : Inport
  Rotation : Inport  Port=2
  Scale : Inport  Port=3
  " Multiport Switch" : MultiPortSwitch
  Display : Display
  Idx : Constant
  wires:
  " Multiport Switch"/1 -> Display/1
  Idx/1 -> " Multiport Switch"/1
  Scale/1 -> " Multiport Switch"/4
  Translation/1 -> " Multiport Switch"/2
  Rotation/1 -> " Multiport Switch"/3

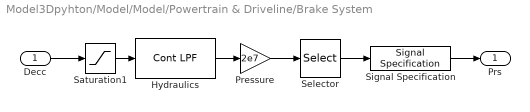
== system Model3Dpyhton/Model/Model/Powertrain & Driveline/Brake System ==
  Decc : Inport
  Hydraulics : autolibutils/Cont LPF  wc=30*pi*2  aMode=2
      settings: SourceProductBaseCode=PW,MT,VE,VP
  Pressure : Gain  Gain=2e7
  Saturation1 : Saturate  UpperLimit=inf  LowerLimit=0  ZeroCross=off
  Selector : Selector  InputPortWidth=1  IndexOptions=Index vector (dialog)  Indices=[1 1 1 1]  OutputSizes=1
  Signal Specification : SignalSpecification  Unit=Pa
  Prs : Outport  VectorParamsAs1DForOutWhenUnconnected=off
  wires:
  Pressure/1 -> Selector/1
  Hydraulics/1 -> Pressure/1
  Saturation1/1 -> Hydraulics/1
  Selector/1 -> Signal Specification/1
  Decc/1 -> Saturation1/1
  Signal Specification/1 -> Prs/1
